simulink model "DIPC"  (R2023a)
settings: Solver=VariableStepAuto  StartTime=0.0  StopTime=10  FixedStep=1e-2  RelTol=1e-3
values from neighbouring files (symbols this model uses):
  d_theta1_init = 0    [dipc_parameters.m]
  d_theta2_init = 0    [dipc_parameters.m]
  d_x_init = 0    [dipc_parameters.m]
  K1 = 1/.8    (= 1.25)    [dipc_parameters.m]
  K2 = 1/6    (= 0.166666666667)    [dipc_parameters.m]
  K3 = 1/.6    (= 1.66666666667)    [dipc_parameters.m]
  K4 = 1/2.5    (= 0.4)    [dipc_parameters.m]
  K5 = 1/1.6    (= 0.625)    [dipc_parameters.m]
  K6 = 1/4.5    (= 0.222222222222)    [dipc_parameters.m]
  K7 = 40    [dipc_parameters.m]
  theta1_init = 0.3    [dipc_parameters.m]
  theta2_init = 0.3    [dipc_parameters.m]
  x_init = 0    [dipc_parameters.m]
libraries: fuzblock x1
settings Model: Creator=luand  LastModifiedBy=luand

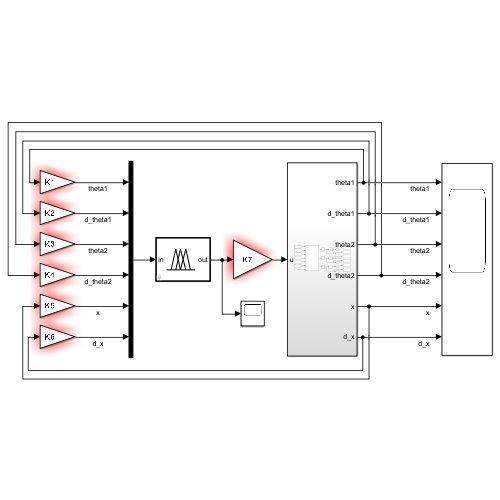
[thumbnail: Simulink's stored preview of the top-level diagram]
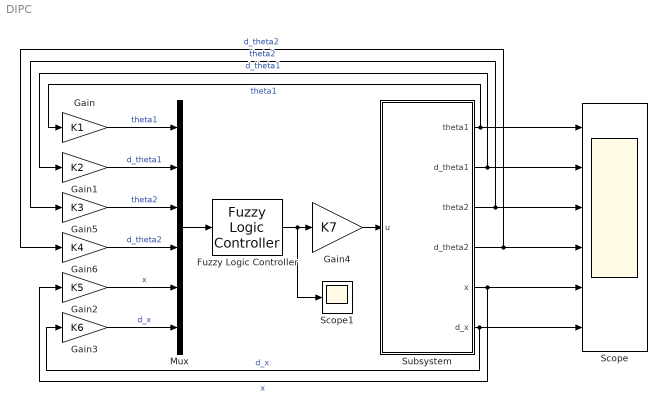
== system DIPC ==
  Fuzzy Logic Controller : fuzblock/Fuzzy Logic  Controller  FIS='fuzzy_dipc_test.fis'  OutputSampleNumber=101  DataType=double  FuzzifiedInputs=off  RuleFiringStrengths=off  RuleOutputs=off  AggregatedOutputs=off  SimulateUsing=Interpreted execution  OutOfRangeInputValueMessage=warning  NoRuleFiredMessage=warning  EmptyOutputFuzzySetMessage=warning
  Gain : Gain  Gain=K1
  Gain1 : Gain  Gain=K2
  Gain2 : Gain  Gain=K5
  Gain3 : Gain  Gain=K6
  Gain4 : Gain  Gain=K7
  Gain5 : Gain  Gain=K3
  Gain6 : Gain  Gain=K4
  Mux : Mux  Inputs=6
  Scope : Scope  NumInputPorts=6
  Scope1 : Scope
  Subsystem : Subsystem
  wires:
  Gain1/1 -> Mux/2  "d_theta1"
  Gain3/1 -> Mux/6  "d_x"
  Gain/1 -> Mux/1  "theta1"
  Fuzzy Logic Controller/1 -> Scope1/1, Gain4/1
  Gain4/1 -> Subsystem/1(u)
  Gain2/1 -> Mux/5  "x"
  Mux/1 -> Fuzzy Logic Controller/1
  Gain5/1 -> Mux/3  "theta2"
  Gain6/1 -> Mux/4  "d_theta2"
  Subsystem/1(theta1) -> Gain/1, Scope/1  "theta1"
  Subsystem/2(d_theta1) -> Gain1/1, Scope/2  "d_theta1"
  Subsystem/3(theta2) -> Gain5/1, Scope/3  "theta2"
  Subsystem/4(d_theta2) -> Gain6/1, Scope/4  "d_theta2"
  Subsystem/5(x) -> Gain2/1, Scope/5  "x"
  Subsystem/6(d_x) -> Gain3/1, Scope/6  "d_x"

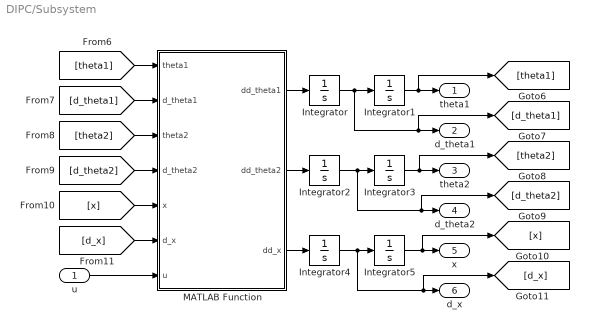
== system DIPC/Subsystem ==
  u : Inport
  Integrator : Integrator  InitialCondition=d_theta1_init
  Integrator1 : Integrator  InitialCondition=theta1_init
  Integrator2 : Integrator  InitialCondition=d_theta2_init
  Integrator3 : Integrator  InitialCondition=theta2_init
  Integrator4 : Integrator  InitialCondition=d_x_init
  Integrator5 : Integrator  InitialCondition=x_init
  MATLAB Function : MATLAB Function  TreatAsAtomicUnit=on
  theta1 : Outport
  d_theta1 : Outport  Port=2
  theta2 : Outport  Port=3
  d_theta2 : Outport  Port=4
  x : Outport  Port=5
  d_x : Outport  Port=6
  wires:
  Integrator1/1 -> theta1/1, [theta1]
  Integrator2/1 -> [d_theta2], d_theta2/1, Integrator3/1
  Integrator3/1 -> [theta2], theta2/1
  Integrator4/1 -> [d_x], d_x/1, Integrator5/1
  Integrator5/1 -> [x], x/1
  MATLAB Function/3(dd_x) -> Integrator4/1
  MATLAB Function/2(dd_theta2) -> Integrator2/1
  MATLAB Function/1(dd_theta1) -> Integrator/1
  u/1 -> MATLAB Function/7(u)
  [d_x] -> MATLAB Function/6(d_x)
  [x] -> MATLAB Function/5(x)
  Integrator/1 -> [d_theta1], d_theta1/1, Integrator1/1
  [theta1] -> MATLAB Function/1(theta1)
  [d_theta1] -> MATLAB Function/2(d_theta1)
  [theta2] -> MATLAB Function/3(theta2)
  [d_theta2] -> MATLAB Function/4(d_theta2)

== matlab function DIPC/Subsystem/MATLAB Function ==
  data: theta1 input; dd_theta1 output; d_theta1 input; theta2 input; d_theta2 input; x input; d_x input; dd_theta2 output; dd_x output; u input
function [dd_theta1,dd_theta2,dd_x] = fcn(theta1,d_theta1,theta2,d_theta2,x,d_x,u)

m0 = 0.8; m1 = 0.5; m2 = 0.3; l1 = 0.3; l2 = 0.3; I1 = 6e-3; I2 = 6e-3; g = 9.81;

% m0 = 1;
% m1 = 0.1;
% m2 = 0.1;
% 
% l1 = 1;
% l2 = 1;
% 
% I1 = 6e-3;
% I2 = 6e-3;
% 
% g = 9.81;

k1 = m0 + m1 + m2;
k2 = m1*l1 + m2*l1;
k3 = m2*l2;
k4 = m1*l1^2 + m2*l1^2 +I1;
k5 = m2*l1*l2;
k6 = m2*l2^2 + I2;

a1 = k1;
a2 = k2*cos(theta1);
a3 = k3*cos(theta2);
A = u+k2*((d_theta1)^2)*sin(theta1)+k3*((d_theta2)^2)*sin(theta2);

b1 = k2*cos(theta1);
b2 = k4;
b3 = k5*cos(theta1-theta2);
B = k2*g*sin(theta1)-k5*sin(theta1-theta2)*((d_theta2)^2);

c1 = k3*cos(theta2);
c2 = k5*cos(theta1-theta2);
c3 = k6;
C = k5*sin(theta1-theta2)*((d_theta1)^2)+k3*g*sin(theta2);

% dd_theta2 = ((C*a1/c1-A)*(b2*a1/b1-a2)/(c2*a1/c1-a2)-(B*a1/b1-A))/...
%             ((c3*a1/c1-c3)*(b2*a1/b1-a2)/(c1*a1/c1-a2)-(b3*a1/b1-a3));
% dd_theta1 = (B*a1/b1-A-(b3*a1/b1-a3)*dd_theta2)/(b2*a1/b1-a2);
% dd_x = (A-a3*dd_theta2-a2*dd_theta1)/a1;

dd_theta2 = (A*b1*c2 - A*b2*c1 - B*a1*c2 + B*a2*c1 + C*a1*b2 - C*a2*b1) /...
            (a1*b2*c3 - a1*b3*c2 - a2*b1*c3 + a2*b3*c1 + a3*b1*c2 - a3*b2*c1);

dd_theta1 = -(A*b1*c3 - A*b3*c1 - B*a1*c3 + B*a3*c1 + C*a1*b3 - C*a3*b1)/...
            (a1*b2*c3 - a1*b3*c2 - a2*b1*c3 + a2*b3*c1 + a3*b1*c2 - a3*b2*c1);

dd_x      = (A*b2*c3 - A*b3*c2 - B*a2*c3 + B*a3*c2 + C*a2*b3 - C*a3*b2) /...
            (a1*b2*c3 - a1*b3*c2 - a2*b1*c3 + a2*b3*c1 + a3*b1*c2 - a3*b2*c1);
